simulink model "Example_8_8"  (R2014a)
settings: Solver=FixedStepDiscrete  SolverMode=SingleTasking  StartTime=0.0  StopTime=10  RelTol=1e-3
libraries: dspsrcs4 x1, dsparch4 x1
settings Model: Creator=Lee Edwards  LastModifiedBy=Lee
settings DataIOCC: SignalLoggingSaveFormat=ModelDataLogs  SaveOutput=off  SignalLogging=off  SaveTime=off
settings OptimizationCC: ExpressionDepthLimit=2147483647
settings DebuggingCC: AlgebraicLoopMsg=error  UnderspecifiedInitializationDetection=Classic  SingleTaskRateTransMsg=error  FcnCallInpInsideContextMsg=UseLocalSettings  StateNameClashWarn=warning
settings GRTTargetCC: CombineOutputUpdateFcns=off  GRTInterface=on

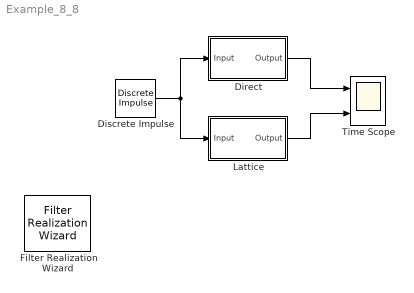
== system Example_8_8 ==
  Direct : Subsystem  Tag=FilterWizardSubSystem
      settings: ErrorFcn=dspFilterRealizedInBasicElemsAlgLoopErrFcnCallback
  Discrete Impulse : dspsrcs4/Discrete  Impulse  Delay=0  SampleTime=1  FrameSample=1  dataType=double  isSigned=on  wordLen=16  udDataType=sfix(16)  fracBitsMode=Best precision  numFracBits=15  OutDataTypeStr=double  LastOutDataTypeStr=double
  Filter Realization Wizard : dsparch4/Filter Realization Wizard
  Lattice : Subsystem  Tag=FilterWizardSubSystem
      settings: ErrorFcn=dspFilterRealizedInBasicElemsAlgLoopErrFcnCallback
  Time Scope : Scope  NumInputPorts=2
      settings: YMin=-2~-2  YMax=3~2  DataFormat=Structure
  wires:
  Discrete Impulse/1 -> Direct/1(Input), Lattice/1(Input)
  Direct/1(Output) -> Time Scope/1
  Lattice/1(Output) -> Time Scope/2

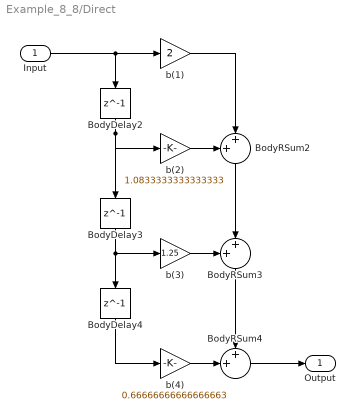
== system Example_8_8/Direct ==
  Input : Inport
  BodyDelay2 : Delay  DelayLength=1  InputProcessing=Inherited
  BodyDelay3 : Delay  DelayLength=1  InputProcessing=Inherited
  BodyDelay4 : Delay  DelayLength=1  InputProcessing=Inherited
  BodyRSum2 : Sum  Inputs=++|  RndMeth=Nearest  SaturateOnIntegerOverflow=on  OutDataTypeStr=Inherit: Same as first input
  BodyRSum3 : Sum  Inputs=++|  RndMeth=Nearest  SaturateOnIntegerOverflow=on  OutDataTypeStr=Inherit: Same as first input
  BodyRSum4 : Sum  Inputs=++|  RndMeth=Nearest  SaturateOnIntegerOverflow=on  OutDataTypeStr=Inherit: Same as first input
  b(1) : Gain  Gain=2  ParamDataTypeStr=float('double')  RndMeth=Nearest  SaturateOnIntegerOverflow=on  OutDataTypeStr=Inherit: Same as input
  b(2) : Gain  Gain=1.0833333333333333  ParamDataTypeStr=float('double')  RndMeth=Nearest  SaturateOnIntegerOverflow=on  OutDataTypeStr=Inherit: Same as input
  b(3) : Gain  Gain=1.25  ParamDataTypeStr=float('double')  RndMeth=Nearest  SaturateOnIntegerOverflow=on  OutDataTypeStr=Inherit: Same as input
  b(4) : Gain  Gain=0.66666666666666663  ParamDataTypeStr=float('double')  RndMeth=Nearest  SaturateOnIntegerOverflow=on  OutDataTypeStr=Inherit: Same as input
  Output : Outport
  wires:
  b(1)/1 -> BodyRSum2/2
  Input/1 -> b(1)/1, BodyDelay2/1
  BodyDelay2/1 -> b(2)/1, BodyDelay3/1
  b(2)/1 -> BodyRSum2/1
  BodyRSum2/1 -> BodyRSum3/2
  BodyDelay3/1 -> b(3)/1, BodyDelay4/1
  b(3)/1 -> BodyRSum3/1
  BodyRSum3/1 -> BodyRSum4/1
  BodyDelay4/1 -> b(4)/1
  b(4)/1 -> BodyRSum4/2
  BodyRSum4/1 -> Output/1

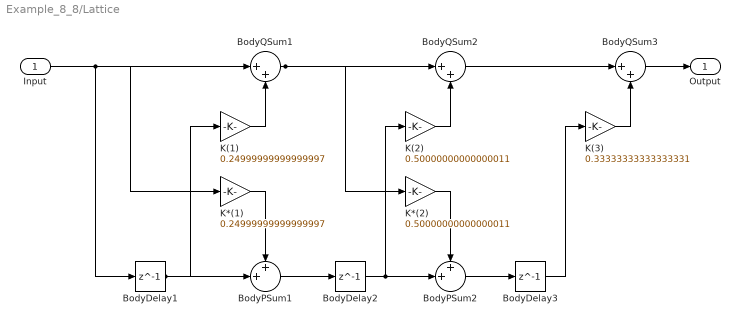
== system Example_8_8/Lattice ==
  Input : Inport
  BodyDelay1 : Delay  DelayLength=1  InputProcessing=Inherited
  BodyDelay2 : Delay  DelayLength=1  InputProcessing=Inherited
  BodyDelay3 : Delay  DelayLength=1  InputProcessing=Inherited
  BodyPSum1 : Sum  Inputs=++|  RndMeth=Nearest  SaturateOnIntegerOverflow=on  OutDataTypeStr=Inherit: Same as first input
  BodyPSum2 : Sum  Inputs=++|  RndMeth=Nearest  SaturateOnIntegerOverflow=on  OutDataTypeStr=Inherit: Same as first input
  BodyQSum1 : Sum  Inputs=|++  RndMeth=Nearest  SaturateOnIntegerOverflow=on  OutDataTypeStr=Inherit: Same as first input
  BodyQSum2 : Sum  Inputs=|++  RndMeth=Nearest  SaturateOnIntegerOverflow=on  OutDataTypeStr=Inherit: Same as first input
  BodyQSum3 : Sum  Inputs=|++  RndMeth=Nearest  SaturateOnIntegerOverflow=on  OutDataTypeStr=Inherit: Same as first input
  K(1) : Gain  Gain=0.24999999999999997  ParamDataTypeStr=float('double')  RndMeth=Nearest  SaturateOnIntegerOverflow=on  OutDataTypeStr=Inherit: Same as input
  K(2) : Gain  Gain=0.50000000000000011  ParamDataTypeStr=float('double')  RndMeth=Nearest  SaturateOnIntegerOverflow=on  OutDataTypeStr=Inherit: Same as input
  K(3) : Gain  Gain=0.33333333333333331  ParamDataTypeStr=float('double')  RndMeth=Nearest  SaturateOnIntegerOverflow=on  OutDataTypeStr=Inherit: Same as input
  K*(1) : Gain  Gain=0.24999999999999997  ParamDataTypeStr=float('double')  RndMeth=Nearest  SaturateOnIntegerOverflow=on  OutDataTypeStr=Inherit: Same as input
  K*(2) : Gain  Gain=0.50000000000000011  ParamDataTypeStr=float('double')  RndMeth=Nearest  SaturateOnIntegerOverflow=on  OutDataTypeStr=Inherit: Same as input
  Output : Outport
  wires:
  BodyQSum1/1 -> BodyQSum2/1, K*(2)/1
  K(1)/1 -> BodyQSum1/2
  K*(1)/1 -> BodyPSum1/1
  BodyPSum1/1 -> BodyDelay2/1
  BodyDelay1/1 -> K(1)/1, BodyPSum1/2
  Input/1 -> BodyQSum1/1, K*(1)/1, BodyDelay1/1
  BodyQSum2/1 -> BodyQSum3/1
  K(2)/1 -> BodyQSum2/2
  K*(2)/1 -> BodyPSum2/1
  BodyPSum2/1 -> BodyDelay3/1
  BodyDelay2/1 -> K(2)/1, BodyPSum2/2
  BodyQSum3/1 -> Output/1
  K(3)/1 -> BodyQSum3/2
  BodyDelay3/1 -> K(3)/1
